simulink model "simulink_interface"  (Simulink 7.8)
settings: Solver=ode45  StartTime=0.0  StopTime=inf  RelTol=1e-3
libraries: etargetslib x7, dspnetwork x6, instrumentlib x3
settings Model: Creator=zev  LastModifiedBy=zev
settings DataIOCC: SignalLoggingSaveFormat=Dataset
settings OptimizationCC: ExpressionDepthLimit=128
settings DebuggingCC: UnderspecifiedInitializationDetection=Simplified  MergeDetectMultiDrivingBlocksExec=error  SolverPrmCheckMsg=none  FrameProcessingCompatibilityMsg=error  StateNameClashWarn=none
settings CodeAppCC: CustomSymbolStrType=$N$R$M_T
settings GRTTargetCC: TargetFunctionLibrary=NOT IN USE  CombineOutputUpdateFcns=on  CPPClassGenCompliant=on

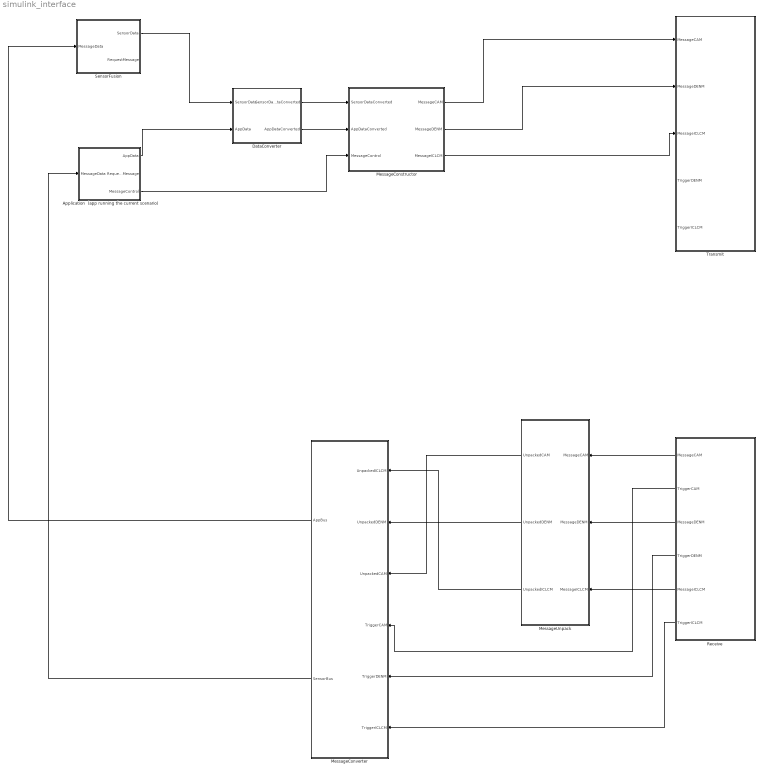
== system simulink_interface ==
  Application  (app running the current scenario) : Subsystem
  DataConverter : Subsystem
  MessageConstructor : Subsystem
  MessageConverter : Subsystem
  MessageUnpack : Subsystem
  Receive : Subsystem
  SensorFusion : Subsystem
  Transmit : Subsystem
  wires:
  Application  (app running the current scenario)/1(AppData) -> DataConverter/2(AppData)
  DataConverter/2(AppDataConverted) -> MessageConstructor/2(AppDataConverted)
  SensorFusion/1(SensorData) -> DataConverter/1(SensorData)
  DataConverter/1(SensorDataConverted) -> MessageConstructor/1(SensorDataConverted)
  MessageConstructor/1(MessageCAM) -> Transmit/1(MessageCAM)
  MessageConstructor/2(MessageDENM) -> Transmit/2(MessageDENM)
  MessageConstructor/3(MessageICLCM) -> Transmit/3(MessageICLCM)
  Application  (app running the current scenario)/3(MessageControl) -> MessageConstructor/3(MessageControl)
  Receive/1(MessageCAM) -> MessageUnpack/1(MessageCAM)
  Receive/2(TriggerCAM) -> MessageConverter/4(TriggerCAM)
  Receive/3(MessageDENM) -> MessageUnpack/2(MessageDENM)
  Receive/4(TriggerDENM) -> MessageConverter/5(TriggerDENM)
  Receive/5(MessageICLCM) -> MessageUnpack/3(MessageICLCM)
  Receive/6(TriggerICLCM) -> MessageConverter/6(TriggerICLCM)
  MessageUnpack/1(UnpackedCAM) -> MessageConverter/3(UnpackedCAM)
  MessageUnpack/2(UnpackedDENM) -> MessageConverter/2(UnpackedDENM)
  MessageConverter/1(AppBus) -> SensorFusion/1(MessageData)
  MessageConverter/2(SensorBus) -> Application  (app running the current scenario)/1(MessageData)
  MessageUnpack/3(UnpackedICLCM) -> MessageConverter/1(UnpackedICLCM)

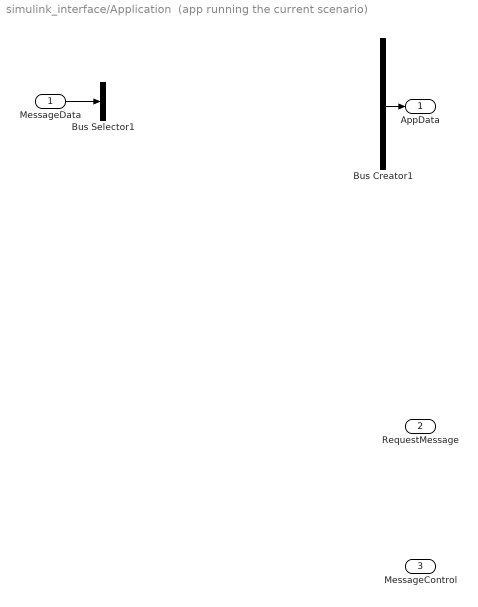
== system simulink_interface/Application  (app running the current scenario) ==
  MessageData : Inport
  Bus Creator1 : BusCreator  Inputs=26
  Bus Selector1 : BusSelector  OutputSignals=StationID,GenerationDeltaTime
  AppData : Outport
  RequestMessage : Outport  Port=2
  MessageControl : Outport  Port=3
  wires:
  MessageData/1 -> Bus Selector1/1
  Bus Creator1/1 -> AppData/1
  ? -> Bus Creator1/1  "DetectionTime"
  ? -> Bus Creator1/2  "CauseCode"
  ? -> Bus Creator1/3  "SubCauseCode"
  ? -> Bus Creator1/4  "ControllerType"
  ? -> Bus Creator1/5  "TargetLongAcc"
  ? -> Bus Creator1/6  "TimeHeadway"
  ? -> Bus Creator1/7  "CruiseSpeed"
  ? -> Bus Creator1/8  "ParticipantsReady"
  ? -> Bus Creator1/9  "StartPlatoon"
  ? -> Bus Creator1/10  "EndOfScenario"
  ? -> Bus Creator1/11  "MioId"
  ? -> Bus Creator1/12  "MioRange"
  ? -> Bus Creator1/13  "MioBearing"
  ? -> Bus Creator1/14  "MioRangeRate"
  ? -> Bus Creator1/15  "Lane"
  ? -> Bus Creator1/16  "ForwardId"
  ? -> Bus Creator1/17  "BackwardId"
  ? -> Bus Creator1/18  "MergeRequest"
  ? -> Bus Creator1/19  "SafeToMerge"
  ? -> Bus Creator1/20  "Flag"
  ? -> Bus Creator1/21  "FlagTail"
  ? -> Bus Creator1/22  "FlagHead"
  ? -> Bus Creator1/23  "PlatoonId"
  ? -> Bus Creator1/24  "DistanceTravelledCz"
  ? -> Bus Creator1/25  "Intention"
  ? -> Bus Creator1/26  "Counter"

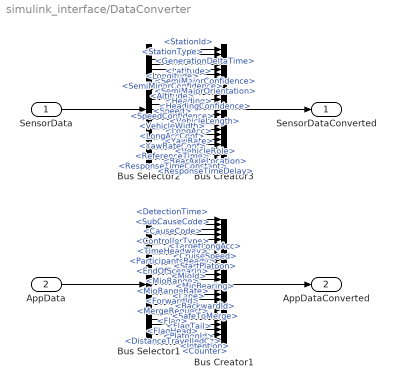
== system simulink_interface/DataConverter ==
  SensorData : Inport
  AppData : Inport  Port=2
  Bus Creator1 : BusCreator  Inputs=26
  Bus Creator3 : BusCreator  Inputs=24
  Bus Selector1 : BusSelector  OutputSignals=DetectionTime,CauseCode,SubCauseCode,ControllerType,TargetLongAcc,TimeHeadway,CruiseSpeed,ParticipantsReady,StartPlatoon,EndOfScenario,MioId,MioRange,MioBearing,MioRangeRate,Lane,ForwardId,BackwardId,MergeRequest,SafeToMerge,Flag,FlagTail,FlagHead,PlatoonId,DistanceTravelledCz,Intention,Counter
  Bus Selector2 : BusSelector  OutputSignals=StationId,GenerationDeltaTime,StationType,Latitude,Longitude,SemiMajorConfidence,SemiMinorConfidence,SemiMajorOrientation,Altitude,Heading,HeadingConfidence,Speed,SpeedConfidence,VehicleLength,VehicleWidth,LongAcc,LongAccConf,YawRate,YawRateConf,VehicleRole,ReferenceTime,RearAxleLocation,ResponseTimeConstant,ResponseTimeDelay
  SensorDataConverted : Outport
  AppDataConverted : Outport  Port=2
  wires:
  Bus Creator3/1 -> SensorDataConverted/1
  SensorData/1 -> Bus Selector2/1
  Bus Selector2/1 -> Bus Creator3/1  "<StationId>"
  Bus Selector2/2 -> Bus Creator3/2  "<GenerationDeltaTime>"
  Bus Selector2/3 -> Bus Creator3/3  "<StationType>"
  Bus Selector2/4 -> Bus Creator3/4  "<Latitude>"
  Bus Selector2/5 -> Bus Creator3/5  "<Longitude>"
  Bus Selector2/6 -> Bus Creator3/6  "<SemiMajorConfidence>"
  Bus Selector2/7 -> Bus Creator3/7  "<SemiMinorConfidence>"
  Bus Selector2/8 -> Bus Creator3/8  "<SemiMajorOrientation>"
  Bus Selector2/9 -> Bus Creator3/9  "<Altitude>"
  Bus Selector2/10 -> Bus Creator3/10  "<Heading>"
  Bus Selector2/11 -> Bus Creator3/11  "<HeadingConfidence>"
  Bus Selector2/12 -> Bus Creator3/12  "<Speed>"
  Bus Selector2/13 -> Bus Creator3/13  "<SpeedConfidence>"
  Bus Selector2/14 -> Bus Creator3/14  "<VehicleLength>"
  Bus Selector2/15 -> Bus Creator3/15  "<VehicleWidth>"
  Bus Selector2/16 -> Bus Creator3/16  "<LongAcc>"
  Bus Selector2/17 -> Bus Creator3/17  "<LongAccConf>"
  Bus Selector2/18 -> Bus Creator3/18  "<YawRate>"
  Bus Selector2/19 -> Bus Creator3/19  "<YawRateConf>"
  Bus Selector2/20 -> Bus Creator3/20  "<VehicleRole>"
  Bus Selector2/21 -> Bus Creator3/21  "<ReferenceTime>"
  Bus Selector2/22 -> Bus Creator3/22  "<RearAxleLocation>"
  Bus Selector2/23 -> Bus Creator3/23  "<ResponseTimeConstant>"
  Bus Selector2/24 -> Bus Creator3/24  "<ResponseTimeDelay>"
  Bus Creator1/1 -> AppDataConverted/1
  AppData/1 -> Bus Selector1/1
  Bus Selector1/1 -> Bus Creator1/1  "<DetectionTime>"
  Bus Selector1/2 -> Bus Creator1/2  "<CauseCode>"
  Bus Selector1/3 -> Bus Creator1/3  "<SubCauseCode>"
  Bus Selector1/4 -> Bus Creator1/4  "<ControllerType>"
  Bus Selector1/5 -> Bus Creator1/5  "<TargetLongAcc>"
  Bus Selector1/6 -> Bus Creator1/6  "<TimeHeadway>"
  Bus Selector1/7 -> Bus Creator1/7  "<CruiseSpeed>"
  Bus Selector1/8 -> Bus Creator1/8  "<ParticipantsReady>"
  Bus Selector1/9 -> Bus Creator1/9  "<StartPlatoon>"
  Bus Selector1/10 -> Bus Creator1/10  "<EndOfScenario>"
  Bus Selector1/11 -> Bus Creator1/11  "<MioId>"
  Bus Selector1/12 -> Bus Creator1/12  "<MioRange>"
  Bus Selector1/13 -> Bus Creator1/13  "<MioBearing>"
  Bus Selector1/14 -> Bus Creator1/14  "<MioRangeRate>"
  Bus Selector1/15 -> Bus Creator1/15  "<Lane>"
  Bus Selector1/16 -> Bus Creator1/16  "<ForwardId>"
  Bus Selector1/17 -> Bus Creator1/17  "<BackwardId>"
  Bus Selector1/18 -> Bus Creator1/18  "<MergeRequest>"
  Bus Selector1/19 -> Bus Creator1/19  "<SafeToMerge>"
  Bus Selector1/20 -> Bus Creator1/20  "<Flag>"
  Bus Selector1/21 -> Bus Creator1/21  "<FlagTail>"
  Bus Selector1/22 -> Bus Creator1/22  "<FlagHead>"
  Bus Selector1/23 -> Bus Creator1/23  "<PlatoonId>"
  Bus Selector1/24 -> Bus Creator1/24  "<DistanceTravelledCz>"
  Bus Selector1/25 -> Bus Creator1/25  "<Intention>"
  Bus Selector1/26 -> Bus Creator1/26  "<Counter>"

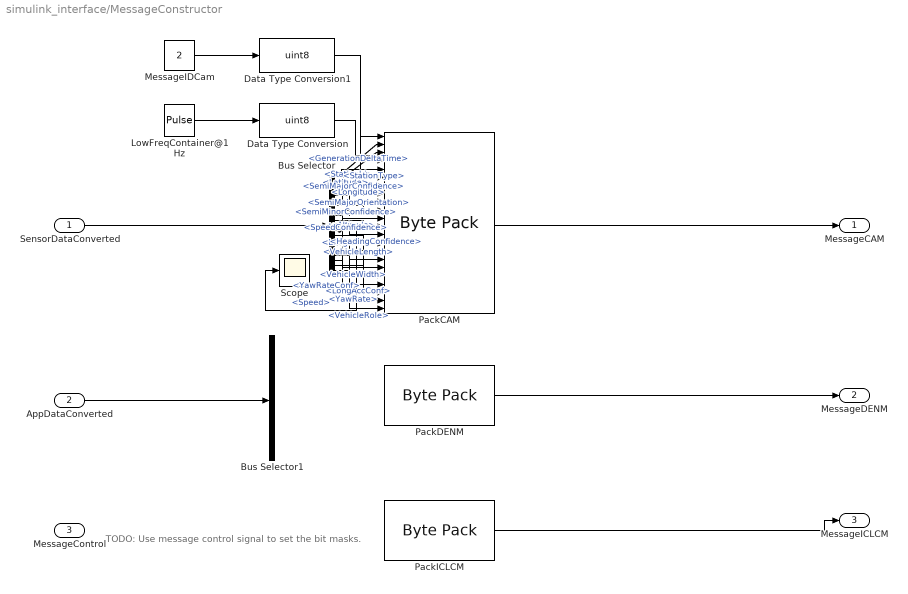
== system simulink_interface/MessageConstructor ==
  note: TODO: Use message control signal to set the bit masks.
  SensorDataConverted : Inport
  AppDataConverted : Inport  Port=2
  MessageControl : Inport  Port=3
  Bus Selector : BusSelector  OutputSignals=StationId,GenerationDeltaTime,StationType,Latitude,Longitude,SemiMajorConfidence,SemiMinorConfidence,SemiMajorOrientation,Altitude,Heading,HeadingConfidence,Speed,SpeedConfidence,VehicleLength,VehicleWidth,LongAcc,LongAccConf,YawRate,YawRateConf,VehicleRole
  Bus Selector1 : BusSelector  OutputSignals=DetectionTime,CauseCode,SubCauseCode,ControllerType,TargetLongAcc,TimeHeadway,CruiseSpeed,ParticipantsReady,StartPlatoon,EndOfScenario,MioId,MioRange,MioBearing,MioRangeRate,Lane,ForwardId,BackwardId,MergeRequest,SafeToMerge,Flag,FlagTail,FlagHead,PlatoonId,DistanceTravelledCz,Intention,Counter
  Data Type Conversion : DataTypeConversion  OutDataTypeStr=uint8
  Data Type Conversion1 : DataTypeConversion  OutDataTypeStr=uint8
  LowFreqContainer@1Hz : DiscretePulseGenerator  PulseType=Time based  Amplitude=128  Period=1  PulseWidth=0.04
  MessageIDCam : Constant  Value=2
  PackCAM : etargetslib/Byte Pack  datatypes={'uint8','int32', 'int32','uint8','int32', 'int32','int32', 'int32','int32', 'int32','int32', 'int32','int32', 'int32','int32', 'int32','int32', 'int32','int32', 'int32','int32', 'int32',}  byteAlign=1
  PackDENM : etargetslib/Byte Pack  datatypes={'int32', 'int32'}  byteAlign=1
  PackICLCM : etargetslib/Byte Pack  datatypes={'int32', 'int32'}  byteAlign=1
  Scope : Scope
      settings: SaveName=ScopeData2  DataFormat=Array
  MessageCAM : Outport
  MessageDENM : Outport  Port=2
  MessageICLCM : Outport  Port=3
  wires:
  Bus Selector/8 -> PackCAM/10  "<SemiMajorOrientation>"
  Bus Selector/4 -> PackCAM/6  "<Latitude>"
  Bus Selector/2 -> PackCAM/3  "<GenerationDeltaTime>"
  Bus Selector/9 -> PackCAM/11  "<Altitude>"
  Bus Selector/6 -> PackCAM/8  "<SemiMajorConfidence>"
  Bus Selector/7 -> PackCAM/9  "<SemiMinorConfidence>"
  Bus Selector/1 -> PackCAM/2  "<StationId>"
  PackCAM/1 -> MessageCAM/1
  Bus Selector/3 -> PackCAM/5  "<StationType>"
  Data Type Conversion/1 -> PackCAM/4
  MessageIDCam/1 -> Data Type Conversion1/1
  Bus Selector/5 -> PackCAM/7  "<Longitude>"
  Bus Selector/15 -> PackCAM/17  "<VehicleWidth>"
  Bus Selector/10 -> PackCAM/12  "<Heading>"
  Bus Selector/16 -> PackCAM/18  "<LongAcc>"
  Bus Selector/12 -> Scope/1, PackCAM/14  "<Speed>"
  Bus Selector/17 -> PackCAM/19  "<LongAccConf>"
  Bus Selector/11 -> PackCAM/13  "<HeadingConfidence>"
  Bus Selector/14 -> PackCAM/16  "<VehicleLength>"
  Bus Selector/13 -> PackCAM/15  "<SpeedConfidence>"
  SensorDataConverted/1 -> Bus Selector/1
  Data Type Conversion1/1 -> PackCAM/1
  Bus Selector/19 -> PackCAM/21  "<YawRateConf>"
  Bus Selector/20 -> PackCAM/22  "<VehicleRole>"
  LowFreqContainer@1Hz/1 -> Data Type Conversion/1
  Bus Selector/18 -> PackCAM/20  "<YawRate>"
  PackDENM/1 -> MessageDENM/1
  AppDataConverted/1 -> Bus Selector1/1
  PackICLCM/1 -> MessageICLCM/1

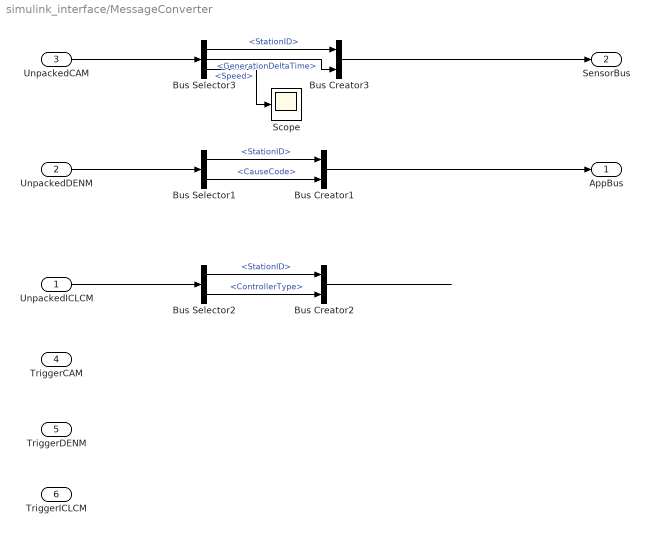
== system simulink_interface/MessageConverter ==
  UnpackedICLCM : Inport
  UnpackedDENM : Inport  Port=2
  UnpackedCAM : Inport  Port=3
  TriggerCAM : Inport  Port=4
  TriggerDENM : Inport  Port=5
  TriggerICLCM : Inport  Port=6
  Bus Creator1 : BusCreator  Inputs=2
  Bus Creator2 : BusCreator  Inputs=2
  Bus Creator3 : BusCreator  Inputs=2
  Bus Selector1 : BusSelector  OutputSignals=StationID,CauseCode
  Bus Selector2 : BusSelector  OutputSignals=StationID,ControllerType
  Bus Selector3 : BusSelector  OutputSignals=StationID,GenerationDeltaTime,Speed
  Scope : Scope
      settings: YMin=0  YMax=1.7e+07  DataFormat=Array
  AppBus : Outport
  SensorBus : Outport  Port=2
  wires:
  Bus Selector2/1 -> Bus Creator2/1  "<StationID>"
  UnpackedICLCM/1 -> Bus Selector2/1
  Bus Selector2/2 -> Bus Creator2/2  "<ControllerType>"
  Bus Creator2/1 -> ?
  Bus Selector1/1 -> Bus Creator1/1  "<StationID>"
  UnpackedDENM/1 -> Bus Selector1/1
  Bus Selector1/2 -> Bus Creator1/2  "<CauseCode>"
  Bus Creator1/1 -> AppBus/1
  Bus Selector3/1 -> Bus Creator3/1  "<StationID>"
  UnpackedCAM/1 -> Bus Selector3/1
  Bus Selector3/2 -> Bus Creator3/2  "<GenerationDeltaTime>"
  Bus Creator3/1 -> SensorBus/1
  Bus Selector3/3 -> Scope/1  "<Speed>"

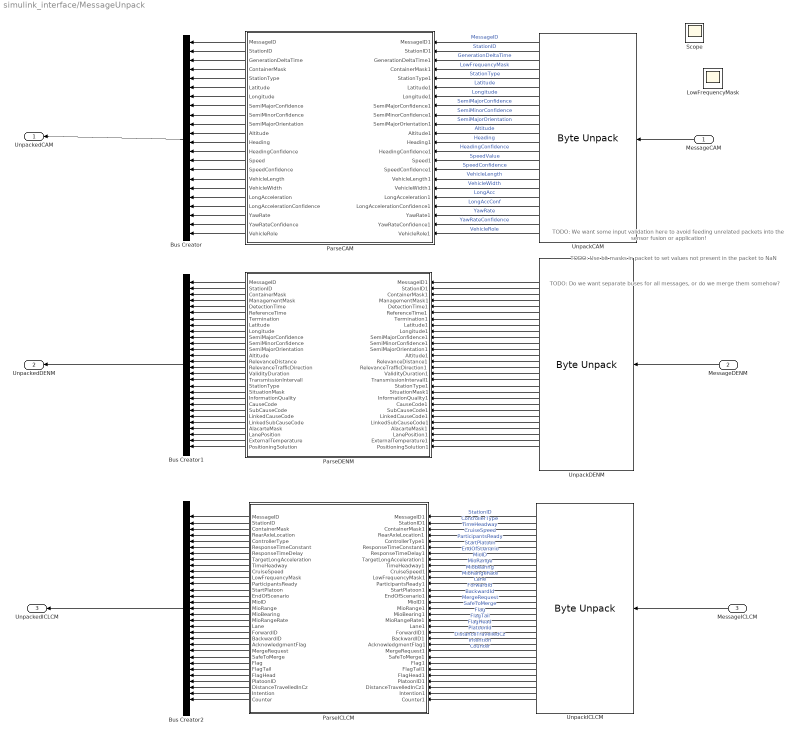
== system simulink_interface/MessageUnpack ==
  note: TODO: Do we want separate buses for all messages, or do we merge them somehow?
  note: TODO: Use bit masks in packet to set values not present in the packet to NaN
  note: TODO: We want some input validation here to avoid feeding unrelated packets
      | into the sensor fusion or application!
  MessageCAM : Inport
  MessageDENM : Inport  Port=2
  MessageICLCM : Inport  Port=3
  Bus Creator : BusCreator  Inputs=22
  Bus Creator1 : BusCreator  Inputs=28
  Bus Creator2 : BusCreator  Inputs=31
  LowFrequencyMask : Scope
      settings: DataFormat=Array
  ParseCAM : MATLAB Function  TreatAsAtomicUnit=on
  ParseDENM : MATLAB Function  TreatAsAtomicUnit=on
  ParseICLCM : MATLAB Function  TreatAsAtomicUnit=on
  Scope : Scope
      settings: SaveName=ScopeData3  DataFormat=Array
  UnpackCAM : etargetslib/Byte Unpack  dimensions={[1],[1],[1],[1],[1],[1],[1],[1],[1],[1],[1],[1],[1],[1],[1],[1],[1],[1],[1],[1],[1],[1],}  datatypes={'uint8','int32', 'int32','uint8','int32', 'int32','int32', 'int32','int32', 'int32','int32', 'int32','int32', 'int32','int32', 'int32','int32', 'int32','int32', 'int32','int32', 'int32',}  byteAlign=1
  UnpackDENM : etargetslib/Byte Unpack  dimensions={[1], [1], [1], [1], [1], [1], [1], [1], [1], [1], [1], [1], [1], [1], [1], [1], [1], [1], [1], [1], [1], [1], [1], [1], [1], [1], [1], [1]}  datatypes="{'uint8', 'int32', 'uint8',  'uint8', 'int32', 'int32', 'int32', 'int32', 'int32',  'int32', 'int32', 'int32', 'int32', 'int32', 'int32', 'int32', 'int32', 'int32', 'uint8',  'int32', 'int32', 'int32', 'int32', 'int32', 'uint8',  'int32', 'int32', 'int32'}"  byteAlign=1
  UnpackICLCM : etargetslib/Byte Unpack  dimensions={[1],[1], [1],[1], [1],[1], [1],[1], [1],[1], [1],[1], [1],[1], [1],[1], [1],[1],[1],[1], [1],[1], [1],[1],[1],[1],[1],[1], [1],[1], [1]}  datatypes={'uint8', 'int32', 'uint8', 'int32', 'int32','int32', 'int32','int32', 'int32','int32', 'uint8', 'int32','int32', 'int32','int32', 'int32','int32', 'int32','int32', 'int32','int32', 'int32','int32', 'int32','int32', 'int32', 'uint32', 'int32','int32', 'int32', 'uint32'}  byteAlign=1
  UnpackedCAM : Outport
  UnpackedDENM : Outport  Port=2
  UnpackedICLCM : Outport  Port=3
  wires:
  UnpackCAM/4 -> ParseCAM/4(ContainerMask1)  "LowFrequencyMask"
  UnpackCAM/10 -> ParseCAM/10(SemiMajorOrientation1)  "SemiMajorOrientation"
  UnpackCAM/11 -> ParseCAM/11(Altitude1)  "Altitude"
  UnpackCAM/9 -> ParseCAM/9(SemiMinorConfidence1)  "SemiMinorConfidence"
  UnpackCAM/7 -> ParseCAM/7(Longitude1)  "Longitude"
  UnpackCAM/8 -> ParseCAM/8(SemiMajorConfidence1)  "SemiMajorConfidence"
  UnpackCAM/6 -> ParseCAM/6(Latitude1)  "Latitude"
  UnpackCAM/5 -> ParseCAM/5(StationType1)  "StationType"
  UnpackCAM/3 -> ParseCAM/3(GenerationDeltaTime1)  "GenerationDeltaTime"
  MessageCAM/1 -> UnpackCAM/1
  MessageDENM/1 -> UnpackDENM/1
  MessageICLCM/1 -> UnpackICLCM/1
  Bus Creator1/1 -> UnpackedDENM/1
  Bus Creator2/1 -> UnpackedICLCM/1
  Bus Creator/1 -> UnpackedCAM/1
  UnpackCAM/2 -> ParseCAM/2(StationID1)  "StationID"
  UnpackCAM/1 -> ParseCAM/1(MessageID1)  "MessageID"
  UnpackCAM/21 -> ParseCAM/21(YawRateConfidence1)  "YawRateConfidence"
  UnpackCAM/22 -> ParseCAM/22(VehicleRole1)  "VehicleRole"
  UnpackCAM/12 -> ParseCAM/12(Heading1)  "Heading"
  UnpackCAM/13 -> ParseCAM/13(HeadingConfidence1)  "HeadingConfidence"
  UnpackCAM/14 -> ParseCAM/14(Speed1)  "SpeedValue"
  UnpackCAM/15 -> ParseCAM/15(SpeedConfidence1)  "SpeedConfidence"
  UnpackCAM/16 -> ParseCAM/16(VehicleLength1)  "VehicleLength"
  UnpackCAM/17 -> ParseCAM/17(VehicleWidth1)  "VehicleWidth"
  UnpackCAM/18 -> ParseCAM/18(LongAcceleration1)  "LongAcc"
  UnpackCAM/19 -> ParseCAM/19(LongAccelerationConfidence1)  "LongAccConf"
  UnpackCAM/20 -> ParseCAM/20(YawRate1)  "YawRate"
  ParseCAM/1(MessageID) -> Bus Creator/1
  ParseCAM/22(VehicleRole) -> Bus Creator/22
  ParseCAM/2(StationID) -> Bus Creator/2
  ParseCAM/3(GenerationDeltaTime) -> Bus Creator/3
  ParseCAM/4(ContainerMask) -> Bus Creator/4
  ParseCAM/5(StationType) -> Bus Creator/5
  ParseCAM/6(Latitude) -> Bus Creator/6
  ParseCAM/7(Longitude) -> Bus Creator/7
  ParseCAM/8(SemiMajorConfidence) -> Bus Creator/8
  ParseCAM/9(SemiMinorConfidence) -> Bus Creator/9
  ParseCAM/10(SemiMajorOrientation) -> Bus Creator/10
  ParseCAM/11(Altitude) -> Bus Creator/11
  ParseCAM/12(Heading) -> Bus Creator/12
  ParseCAM/13(HeadingConfidence) -> Bus Creator/13
  ParseCAM/14(Speed) -> Bus Creator/14
  ParseCAM/15(SpeedConfidence) -> Bus Creator/15
  ParseCAM/16(VehicleLength) -> Bus Creator/16
  ParseCAM/17(VehicleWidth) -> Bus Creator/17
  ParseCAM/18(LongAcceleration) -> Bus Creator/18
  ParseCAM/19(LongAccelerationConfidence) -> Bus Creator/19
  ParseCAM/20(YawRate) -> Bus Creator/20
  ParseCAM/21(YawRateConfidence) -> Bus Creator/21
  UnpackDENM/1 -> ParseDENM/1(MessageID1)
  UnpackDENM/2 -> ParseDENM/2(StationID1)
  UnpackDENM/3 -> ParseDENM/3(ContainerMask1)
  UnpackDENM/4 -> ParseDENM/4(ManagementMask1)
  UnpackDENM/5 -> ParseDENM/5(DetectionTime1)
  UnpackDENM/6 -> ParseDENM/6(ReferenceTime1)
  UnpackDENM/7 -> ParseDENM/7(Termination1)
  UnpackDENM/8 -> ParseDENM/8(Latitude1)
  UnpackDENM/9 -> ParseDENM/9(Longitude1)
  UnpackDENM/10 -> ParseDENM/10(SemiMajorConfidence1)
  UnpackDENM/11 -> ParseDENM/11(SemiMinorConfidence1)
  UnpackDENM/12 -> ParseDENM/12(SemiMajorOrientation1)
  UnpackDENM/13 -> ParseDENM/13(Altitude1)
  UnpackDENM/14 -> ParseDENM/14(RelevanceDistance1)
  UnpackDENM/15 -> ParseDENM/15(RelevanceTrafficDirection1)
  UnpackDENM/16 -> ParseDENM/16(ValidityDuration1)
  UnpackDENM/17 -> ParseDENM/17(TransmissionIntervall1)
  UnpackDENM/18 -> ParseDENM/18(StationType1)
  UnpackDENM/19 -> ParseDENM/19(SituationMask1)
  UnpackDENM/20 -> ParseDENM/20(InformationQuality1)
  UnpackDENM/21 -> ParseDENM/21(CauseCode1)
  UnpackDENM/22 -> ParseDENM/22(SubCauseCode1)
  UnpackDENM/23 -> ParseDENM/23(LinkedCauseCode1)
  UnpackDENM/24 -> ParseDENM/24(LinkedSubCauseCode1)
  UnpackDENM/25 -> ParseDENM/25(AlacarteMask1)
  UnpackDENM/26 -> ParseDENM/26(LanePosition1)
  UnpackDENM/27 -> ParseDENM/27(ExternalTemperature1)
  UnpackDENM/28 -> ParseDENM/28(PositioningSolution1)
  ParseDENM/1(MessageID) -> Bus Creator1/1
  ParseDENM/2(StationID) -> Bus Creator1/2
  ParseDENM/3(ContainerMask) -> Bus Creator1/3
  ParseDENM/4(ManagementMask) -> Bus Creator1/4
  ParseDENM/5(DetectionTime) -> Bus Creator1/5
  ParseDENM/6(ReferenceTime) -> Bus Creator1/6
  ParseDENM/7(Termination) -> Bus Creator1/7
  ParseDENM/8(Latitude) -> Bus Creator1/8
  ParseDENM/9(Longitude) -> Bus Creator1/9
  ParseDENM/10(SemiMajorConfidence) -> Bus Creator1/10
  ParseDENM/11(SemiMinorConfidence) -> Bus Creator1/11
  ParseDENM/12(SemiMajorOrientation) -> Bus Creator1/12
  ParseDENM/13(Altitude) -> Bus Creator1/13
  ParseDENM/14(RelevanceDistance) -> Bus Creator1/14
  ParseDENM/15(RelevanceTrafficDirection) -> Bus Creator1/15
  ParseDENM/16(ValidityDuration) -> Bus Creator1/16
  ParseDENM/17(TransmissionIntervall) -> Bus Creator1/17
  ParseDENM/18(StationType) -> Bus Creator1/18
  ParseDENM/19(SituationMask) -> Bus Creator1/19
  ParseDENM/20(InformationQuality) -> Bus Creator1/20
  ParseDENM/21(CauseCode) -> Bus Creator1/21
  ParseDENM/22(SubCauseCode) -> Bus Creator1/22
  ParseDENM/23(LinkedCauseCode) -> Bus Creator1/23
  ParseDENM/24(LinkedSubCauseCode) -> Bus Creator1/24
  ParseDENM/25(AlacarteMask) -> Bus Creator1/25
  ParseDENM/26(LanePosition) -> Bus Creator1/26
  ParseDENM/27(ExternalTemperature) -> Bus Creator1/27
  ParseDENM/28(PositioningSolution) -> Bus Creator1/28
  UnpackICLCM/1 -> ParseICLCM/1(MessageID1)  "StationID"
  UnpackICLCM/2 -> ParseICLCM/2(StationID1)  "ControllerType"
  UnpackICLCM/3 -> ParseICLCM/3(ContainerMask1)  "TimeHeadway"
  UnpackICLCM/4 -> ParseICLCM/4(RearAxleLocation1)  "CruiseSpeed"
  UnpackICLCM/5 -> ParseICLCM/5(ControllerType1)  "ParticipantsReady"
  UnpackICLCM/6 -> ParseICLCM/6(ResponseTimeConstant1)  "StartPlatoon"
  UnpackICLCM/7 -> ParseICLCM/7(ResponseTimeDelay1)  "EndOfScenario"
  UnpackICLCM/8 -> ParseICLCM/8(TargetLongAcceleration1)  "MioID"
  UnpackICLCM/9 -> ParseICLCM/9(TimeHeadway1)  "MioRange"
  UnpackICLCM/10 -> ParseICLCM/10(CruiseSpeed1)  "MioBearing"
  UnpackICLCM/11 -> ParseICLCM/11(LowFrequencyMask1)  "MioRangeRate"
  UnpackICLCM/12 -> ParseICLCM/12(ParticipantsReady1)  "Lane"
  UnpackICLCM/13 -> ParseICLCM/13(StartPlatoon1)  "ForwardId"
  UnpackICLCM/14 -> ParseICLCM/14(EndOfScenario1)  "BackwardId"
  UnpackICLCM/15 -> ParseICLCM/15(MioID1)  "MergeRequest"
  UnpackICLCM/16 -> ParseICLCM/16(MioRange1)  "SafeToMerge"
  UnpackICLCM/17 -> ParseICLCM/17(MioBearing1)  "Flag"
  UnpackICLCM/18 -> ParseICLCM/18(MioRangeRate1)  "FlagTail"
  UnpackICLCM/19 -> ParseICLCM/19(Lane1)  "FlagHead"
  UnpackICLCM/20 -> ParseICLCM/20(ForwardID1)  "PlatoonId"
  UnpackICLCM/21 -> ParseICLCM/21(BackwardID1)  "DistanceTravelledCz"
  UnpackICLCM/22 -> ParseICLCM/22(AcknowledgmentFlag1)  "Intention"
  UnpackICLCM/23 -> ParseICLCM/23(MergeRequest1)  "Counter"
  UnpackICLCM/24 -> ParseICLCM/24(SafeToMerge1)
  UnpackICLCM/25 -> ParseICLCM/25(Flag1)
  UnpackICLCM/26 -> ParseICLCM/26(FlagTail1)
  UnpackICLCM/27 -> ParseICLCM/27(FlagHead1)
  UnpackICLCM/28 -> ParseICLCM/28(PlatoonID1)
  UnpackICLCM/29 -> ParseICLCM/29(DistanceTravelledInCz1)
  UnpackICLCM/30 -> ParseICLCM/30(Intention1)
  UnpackICLCM/31 -> ParseICLCM/31(Counter1)
  ParseICLCM/1(MessageID) -> Bus Creator2/1
  ParseICLCM/2(StationID) -> Bus Creator2/2
  ParseICLCM/3(ContainerMask) -> Bus Creator2/3
  ParseICLCM/4(RearAxleLocation) -> Bus Creator2/4
  ParseICLCM/5(ControllerType) -> Bus Creator2/5
  ParseICLCM/6(ResponseTimeConstant) -> Bus Creator2/6
  ParseICLCM/7(ResponseTimeDelay) -> Bus Creator2/7
  ParseICLCM/8(TargetLongAcceleration) -> Bus Creator2/8
  ParseICLCM/9(TimeHeadway) -> Bus Creator2/9
  ParseICLCM/10(CruiseSpeed) -> Bus Creator2/10
  ParseICLCM/11(LowFrequencyMask) -> Bus Creator2/11
  ParseICLCM/12(ParticipantsReady) -> Bus Creator2/12
  ParseICLCM/13(StartPlatoon) -> Bus Creator2/13
  ParseICLCM/14(EndOfScenario) -> Bus Creator2/14
  ParseICLCM/15(MioID) -> Bus Creator2/15
  ParseICLCM/16(MioRange) -> Bus Creator2/16
  ParseICLCM/17(MioBearing) -> Bus Creator2/17
  ParseICLCM/18(MioRangeRate) -> Bus Creator2/18
  ParseICLCM/19(Lane) -> Bus Creator2/19
  ParseICLCM/20(ForwardID) -> Bus Creator2/20
  ParseICLCM/21(BackwardID) -> Bus Creator2/21
  ParseICLCM/22(AcknowledgmentFlag) -> Bus Creator2/22
  ParseICLCM/23(MergeRequest) -> Bus Creator2/23
  ParseICLCM/24(SafeToMerge) -> Bus Creator2/24
  ParseICLCM/25(Flag) -> Bus Creator2/25
  ParseICLCM/26(FlagTail) -> Bus Creator2/26
  ParseICLCM/27(FlagHead) -> Bus Creator2/27
  ParseICLCM/28(PlatoonID) -> Bus Creator2/28
  ParseICLCM/29(DistanceTravelledInCz) -> Bus Creator2/29
  ParseICLCM/30(Intention) -> Bus Creator2/30
  ParseICLCM/31(Counter) -> Bus Creator2/31

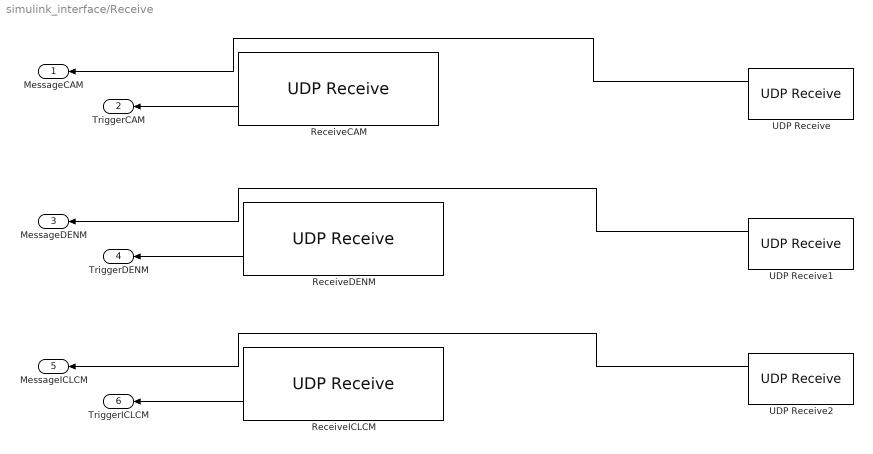
== system simulink_interface/Receive ==
  ReceiveCAM : instrumentlib/UDP Receive  Host=127.0.0.1  Port=4000  LocalPort=-1  DataSize="[1  82]"  EnableBlockingMode=off  Timeout=10  SampleTime=0.01  DataType=uint8  ByteOrder=BigEndian
  ReceiveDENM : instrumentlib/UDP Receive  Host=0.0.0.0  Port=4001  LocalPort=-1  DataSize="[1  12]"  EnableBlockingMode=off  Timeout=10  SampleTime=0.01  DataType=uint8  ByteOrder=BigEndian
  ReceiveICLCM : instrumentlib/UDP Receive  Host=0.0.0.0  Port=4002  LocalPort=-1  DataSize="[1  92]"  EnableBlockingMode=off  Timeout=10  SampleTime=0.01  DataType=uint8  ByteOrder=BigEndian
  UDP Receive : dspnetwork/UDP Receive  localURL='0.0.0.0'  localPort=5000  remoteURL='0.0.0.0'  remotePort=-1  recvBufferSize=8192  dims=82  signalDatatype=uint8  isVarSize=off  showBlockingTime=off  blockingTime=0  sampletime=0.04
  UDP Receive1 : dspnetwork/UDP Receive  localURL='0.0.0.0'  localPort=5001  remoteURL='0.0.0.0'  remotePort=-1  recvBufferSize=8192  dims=97  signalDatatype=uint8  isVarSize=off  showBlockingTime=off  blockingTime=0  sampletime=0.04
  UDP Receive2 : dspnetwork/UDP Receive  localURL='0.0.0.0'  localPort=5002  remoteURL='0.0.0.0'  remotePort=-1  recvBufferSize=8192  dims=115  signalDatatype=uint8  isVarSize=off  showBlockingTime=off  blockingTime=0  sampletime=0.04
  MessageCAM : Outport
  TriggerCAM : Outport  Port=2
  MessageDENM : Outport  Port=3
  TriggerDENM : Outport  Port=4
  MessageICLCM : Outport  Port=5
  TriggerICLCM : Outport  Port=6
  wires:
  UDP Receive/1 -> MessageCAM/1
  ReceiveICLCM/2 -> TriggerICLCM/1
  UDP Receive2/1 -> MessageICLCM/1
  ReceiveDENM/2 -> TriggerDENM/1
  UDP Receive1/1 -> MessageDENM/1
  ReceiveCAM/2 -> TriggerCAM/1

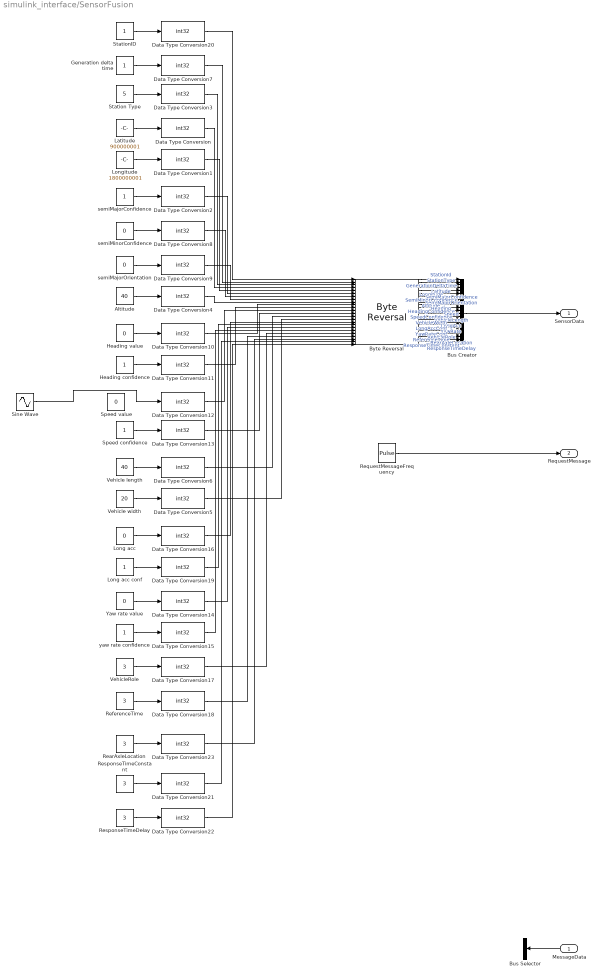
== system simulink_interface/SensorFusion ==
  MessageData : Inport
  Altitude : Constant  Value=40
  Bus Creator : BusCreator  Inputs=24
  Bus Selector : BusSelector  OutputSignals=StationID
  Byte Reversal : etargetslib/Byte Reversal  numInp=24
  Data Type Conversion{,1..23} (24 alike) : DataTypeConversion  OutDataTypeStr=int32
  Generation delta time : Constant
  Heading confidence : Constant
  Heading value : Constant  Value=0
  Latitude : Constant  Value=900000001
  Long acc : Constant  Value=0
  Long acc conf : Constant
  Longitude : Constant  Value=1800000001
  RearAxleLocation : Constant  Value=3
  ReferenceTime : Constant  Value=3
  RequestMessageFrequency : DiscretePulseGenerator  PulseType=Time based  Period=0.01  PulseWidth=5
  ResponseTimeConstant : Constant  Value=3
  ResponseTimeDelay : Constant  Value=3
  Sine Wave : Sin  Bias=1  Frequency=100  SampleTime=0
  Speed confidence : Constant
  Speed value : Constant  Value=0
  Station Type : Constant  Value=5
  StationID : Constant
  Vehicle length : Constant  Value=40
  Vehicle width : Constant  Value=20
  VehicleRole : Constant  Value=3
  Yaw rate value : Constant  Value=0
  "semiMajorConfidence " : Constant
  "semiMajorOrientation " : Constant  Value=0
  "semiMinorConfidence " : Constant  Value=0
  yaw rate confidence : Constant
  SensorData : Outport
  RequestMessage : Outport  Port=2
  wires:
  Bus Creator/1 -> SensorData/1
  Station Type/1 -> Data Type Conversion3/1
  Generation delta time/1 -> Data Type Conversion7/1
  yaw rate confidence/1 -> Data Type Conversion15/1
  Long acc/1 -> Data Type Conversion16/1
  VehicleRole/1 -> Data Type Conversion17/1
  Long acc conf/1 -> Data Type Conversion19/1
  ReferenceTime/1 -> Data Type Conversion18/1
  Vehicle length/1 -> Data Type Conversion6/1
  Vehicle width/1 -> Data Type Conversion5/1
  Latitude/1 -> Data Type Conversion/1
  Longitude/1 -> Data Type Conversion1/1
  "semiMajorConfidence "/1 -> Data Type Conversion2/1
  "semiMinorConfidence "/1 -> Data Type Conversion8/1
  "semiMajorOrientation "/1 -> Data Type Conversion9/1
  Heading confidence/1 -> Data Type Conversion11/1
  Heading value/1 -> Data Type Conversion10/1
  Sine Wave/1 -> Data Type Conversion12/1
  Speed confidence/1 -> Data Type Conversion13/1
  Yaw rate value/1 -> Data Type Conversion14/1
  StationID/1 -> Data Type Conversion20/1
  Altitude/1 -> Data Type Conversion4/1
  ResponseTimeConstant/1 -> Data Type Conversion21/1
  ResponseTimeDelay/1 -> Data Type Conversion22/1
  RearAxleLocation/1 -> Data Type Conversion23/1
  Data Type Conversion20/1 -> Byte Reversal/1
  Data Type Conversion7/1 -> Byte Reversal/2
  Data Type Conversion3/1 -> Byte Reversal/3
  Data Type Conversion/1 -> Byte Reversal/4
  Data Type Conversion1/1 -> Byte Reversal/5
  Data Type Conversion2/1 -> Byte Reversal/6
  Data Type Conversion8/1 -> Byte Reversal/7
  Data Type Conversion9/1 -> Byte Reversal/8
  Data Type Conversion4/1 -> Byte Reversal/9
  Data Type Conversion10/1 -> Byte Reversal/10
  Data Type Conversion11/1 -> Byte Reversal/11
  Data Type Conversion12/1 -> Byte Reversal/12
  Data Type Conversion13/1 -> Byte Reversal/13
  Data Type Conversion6/1 -> Byte Reversal/14
  Data Type Conversion5/1 -> Byte Reversal/15
  Data Type Conversion16/1 -> Byte Reversal/16
  Data Type Conversion19/1 -> Byte Reversal/17
  Data Type Conversion14/1 -> Byte Reversal/18
  Data Type Conversion15/1 -> Byte Reversal/19
  Data Type Conversion17/1 -> Byte Reversal/20
  Data Type Conversion18/1 -> Byte Reversal/21
  Data Type Conversion23/1 -> Byte Reversal/22
  Data Type Conversion21/1 -> Byte Reversal/23
  Data Type Conversion22/1 -> Byte Reversal/24
  Byte Reversal/1 -> Bus Creator/1  "StationId"
  Byte Reversal/2 -> Bus Creator/2  "GenerationDeltaTime"
  Byte Reversal/3 -> Bus Creator/3  "StationType"
  Byte Reversal/4 -> Bus Creator/4  "Latitude"
  Byte Reversal/5 -> Bus Creator/5  "Longitude"
  Byte Reversal/6 -> Bus Creator/6  "SemiMajorConfidence"
  Byte Reversal/7 -> Bus Creator/7  "SemiMinorConfidence"
  Byte Reversal/8 -> Bus Creator/8  "SemiMajorOrientation"
  Byte Reversal/9 -> Bus Creator/9  "Altitude"
  Byte Reversal/10 -> Bus Creator/10  "Heading"
  Byte Reversal/11 -> Bus Creator/11  "HeadingConfidence"
  Byte Reversal/12 -> Bus Creator/12  "Speed"
  Byte Reversal/13 -> Bus Creator/13  "SpeedConfidence"
  Byte Reversal/14 -> Bus Creator/14  "VehicleLength"
  Byte Reversal/15 -> Bus Creator/15  "VehicleWidth"
  Byte Reversal/16 -> Bus Creator/16  "LongAcc"
  Byte Reversal/17 -> Bus Creator/17  "LongAccConf"
  Byte Reversal/18 -> Bus Creator/18  "YawRate"
  Byte Reversal/19 -> Bus Creator/19  "YawRateConf"
  Byte Reversal/20 -> Bus Creator/20  "VehicleRole"
  Byte Reversal/21 -> Bus Creator/21  "ReferenceTime"
  Byte Reversal/22 -> Bus Creator/22  "RearAxleLocation"
  Byte Reversal/23 -> Bus Creator/23  "ResponseTimeConstant"
  Byte Reversal/24 -> Bus Creator/24  "ResponseTimeDelay"
  RequestMessageFrequency/1 -> RequestMessage/1
  MessageData/1 -> Bus Selector/1

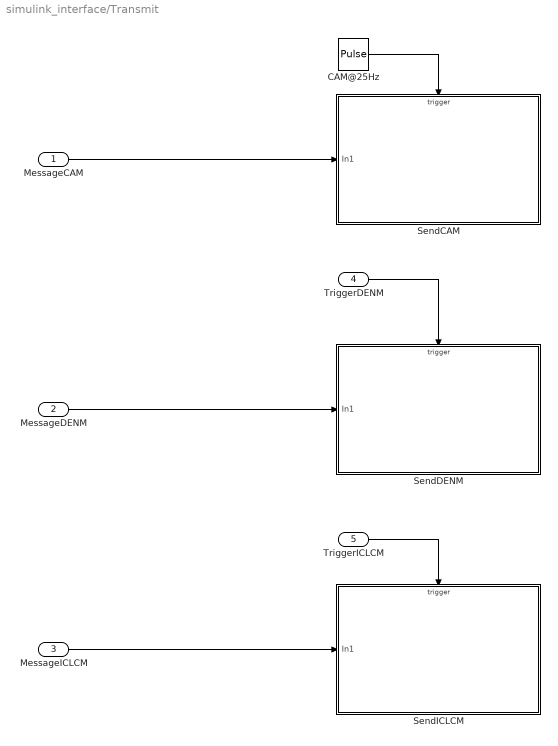
== system simulink_interface/Transmit ==
  MessageCAM : Inport
  MessageDENM : Inport  Port=2
  MessageICLCM : Inport  Port=3
  TriggerDENM : Inport  Port=4
  TriggerICLCM : Inport  Port=5
  CAM@25Hz : DiscretePulseGenerator  PulseType=Time based  Period=0.04  PulseWidth=5
  SendCAM : Subsystem
  SendDENM : Subsystem
  SendICLCM : Subsystem
  wires:
  MessageDENM/1 -> SendDENM/1(In1)
  MessageICLCM/1 -> SendICLCM/1(In1)
  TriggerDENM/1 -> SendDENM/Trigger
  TriggerICLCM/1 -> SendICLCM/Trigger
  CAM@25Hz/1 -> SendCAM/Trigger
  MessageCAM/1 -> SendCAM/1(In1)

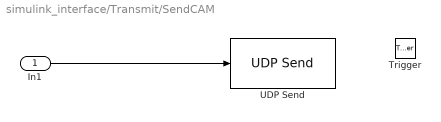
== system simulink_interface/Transmit/SendCAM ==
  In1 : Inport
  Trigger : TriggerPort  PortDimensions=1
  UDP Send : dspnetwork/UDP Send  remoteURL='127.0.0.1'  remotePort=5000  localURL='0.0.0.0'  localPortSource=Automatically determine  localPort=-1  sampletime=-1  separateLengthPort=0
  wires:
  In1/1 -> UDP Send/1

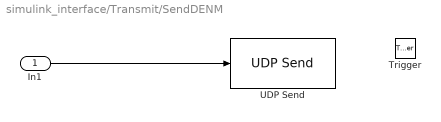
== system simulink_interface/Transmit/SendDENM ==
  In1 : Inport
  Trigger : TriggerPort  PortDimensions=1
  UDP Send : dspnetwork/UDP Send  remoteURL='127.0.0.1'  remotePort=5001  localURL='0.0.0.0'  localPortSource=Automatically determine  localPort=-1  sampletime=-1  separateLengthPort=0
  wires:
  In1/1 -> UDP Send/1

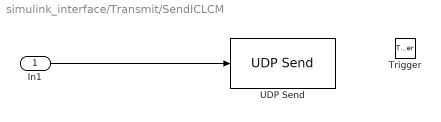
== system simulink_interface/Transmit/SendICLCM ==
  In1 : Inport
  Trigger : TriggerPort  PortDimensions=1
  UDP Send : dspnetwork/UDP Send  remoteURL='127.0.0.1'  remotePort=5001  localURL='0.0.0.0'  localPortSource=Automatically determine  localPort=-1  sampletime=-1  separateLengthPort=0
  wires:
  In1/1 -> UDP Send/1

== matlab function MessageUnpack/ParseDENM ==
  data: MessageID1 input double; MessageID output double; StationID1 input double; ContainerMask1 input double; ManagementMask1 input double; DetectionTime1 input double; ReferenceTime1 input double; Termination1 input double; Latitude1 input double; Longitude1 input double; SemiMajorConfidence1 input double; SemiMinorConfidence1 input double; SemiMajorOrientation1 input double; Altitude1 input double; RelevanceDistance1 input double; RelevanceTrafficDirection1 input double; ValidityDuration1 input double; TransmissionIntervall1 input double; StationType1 input double; SituationMask1 input double; InformationQuality1 input double; CauseCode1 input double; SubCauseCode1 input double; LinkedCauseCode1 input double; LinkedSubCauseCode1 input double; AlacarteMask1 input double; LanePosition1 input double; ExternalTemperature1 input double; PositioningSolution1 input double; StationID output double; ContainerMask output double; ManagementMask output double; DetectionTime output double; ReferenceTime output double; Termination output double; Latitude output double; Longitude output double; SemiMajorConfidence output double; SemiMinorConfidence output double; SemiMajorOrientation output double; Altitude output double; RelevanceDistance output double; RelevanceTrafficDirection output double; ValidityDuration output double; TransmissionIntervall output double; StationType output double; SituationMask output double; InformationQuality output double; CauseCode output double; SubCauseCode output double; LinkedCauseCode output double; LinkedSubCauseCode output double; AlacarteMask output double; LanePosition output double; ExternalTemperature output double; PositioningSolution output double
function [MessageID, StationID, ContainerMask, ManagementMask, DetectionTime, ReferenceTime, Termination, Latitude, Longitude, SemiMajorConfidence, SemiMinorConfidence, SemiMajorOrientation, Altitude, RelevanceDistance, RelevanceTrafficDirection, ValidityDuration, TransmissionIntervall, StationType, SituationMask, InformationQuality, CauseCode, SubCauseCode, LinkedCauseCode, LinkedSubCauseCode, AlacarteMask, LanePosition, ExternalTemperature, PositioningSolution] = parseDENM(MessageID1, StationID1, ContainerMask1, ManagementMask1, DetectionTime1, ReferenceTime1, Termination1, Latitude1, Longitude1, SemiMajorConfidence1, SemiMinorConfidence1, SemiMajorOrientation1, Altitude1, RelevanceDistance1, RelevanceTrafficDirection1, ValidityDuration1, TransmissionIntervall1, StationType1, SituationMask1, InformationQuality1, CauseCode1, SubCauseCode1, LinkedCauseCode1, LinkedSubCauseCode1, AlacarteMask1, LanePosition1, ExternalTemperature1, PositioningSolution1)
%parseDENM - Parses a local DENM message.



MessageID = MessageID1;
StationID = StationID1;
ContainerMask = ContainerMask1;
ManagementMask = ManagementMask1;
DetectionTime = DetectionTime1;
ReferenceTime = ReferenceTime1;
Termination = Termination1;
Latitude = Latitude1;
Longitude = Longitude1; 
SemiMajorConfidence = SemiMajorConfidence1;
SemiMinorConfidence = SemiMinorConfidence1; 
SemiMajorOrientation = SemiMajorOrientation1;
Altitude = Altitude1; 
RelevanceDistance = RelevanceDistance1;
RelevanceTrafficDirection = RelevanceTrafficDirection1; 
ValidityDuration = ValidityDuration1; 
TransmissionIntervall = TransmissionIntervall1; 
StationType = StationType1; 
SituationMask = SituationMask1; 
InformationQuality = InformationQuality1; 
CauseCode = CauseCode1; 
SubCauseCode = SubCauseCode1; 
LinkedCauseCode = LinkedCauseCode1; 
LinkedSubCauseCode = LinkedSubCauseCode1; 
AlacarteMask = AlacarteMask1;
LanePosition = LanePosition1;
ExternalTemperature = ExternalTemperature1; 
PositioningSolution = PositioningSolution1;

== matlab function MessageUnpack/ParseCAM ==
  data: MessageID output double; MessageID1 input double; StationID output double; GenerationDeltaTime output double; ContainerMask output double; StationType output double; Latitude output double; Longitude output double; SemiMajorConfidence output double; SemiMinorConfidence output double; SemiMajorOrientation output double; Altitude output double; Heading output double; HeadingConfidence output double; Speed output double; SpeedConfidence output double; VehicleLength output double; VehicleWidth output double; LongAcceleration output double; LongAccelerationConfidence output double; YawRate output double; YawRateConfidence output double; VehicleRole output double; StationID1 input double; GenerationDeltaTime1 input double; ContainerMask1 input double; StationType1 input double; Latitude1 input double; Longitude1 input double; SemiMajorConfidence1 input double; SemiMinorConfidence1 input double; SemiMajorOrientation1 input double; Altitude1 input double; Heading1 input double; HeadingConfidence1 input double; Speed1 input double; SpeedConfidence1 input double; VehicleLength1 input double; VehicleWidth1 input double; LongAcceleration1 input double; LongAccelerationConfidence1 input double; YawRate1 input double; YawRateConfidence1 input double; VehicleRole1 input double
function [MessageID, StationID, GenerationDeltaTime, ContainerMask, StationType, Latitude, Longitude, SemiMajorConfidence, SemiMinorConfidence, SemiMajorOrientation, Altitude, Heading, HeadingConfidence, Speed, SpeedConfidence, VehicleLength, VehicleWidth, LongAcceleration, LongAccelerationConfidence, YawRate, YawRateConfidence, VehicleRole] = parseCAM(MessageID1, StationID1, GenerationDeltaTime1, ContainerMask1, StationType1, Latitude1, Longitude1, SemiMajorConfidence1, SemiMinorConfidence1, SemiMajorOrientation1, Altitude1, Heading1, HeadingConfidence1, Speed1, SpeedConfidence1, VehicleLength1, VehicleWidth1, LongAcceleration1, LongAccelerationConfidence1, YawRate1, YawRateConfidence1, VehicleRole1)
%parseCAM - Parses a local CAM message. Used to do some conversion in order
%to make the values compatible with the Simulink model.

MessageID = MessageID1;
StationID = StationID1;
GenerationDeltaTime = GenerationDeltaTime1;
ContainerMask = ContainerMask1;
StationType = StationType1;
Latitude = Latitude1;
Longitude = Longitude1;
SemiMajorConfidence = SemiMajorConfidence1;
SemiMinorConfidence = SemiMinorConfidence1;
SemiMajorOrientation = SemiMajorOrientation1;
Altitude = Altitude1;
Heading = Heading1;
HeadingConfidence = HeadingConfidence1;
Speed = Speed1;
SpeedConfidence = SpeedConfidence1;
VehicleLength = VehicleLength1;
VehicleWidth = VehicleWidth1;
LongAcceleration = LongAcceleration1;
LongAccelerationConfidence = LongAccelerationConfidence1;
YawRate = YawRate1;
YawRateConfidence = YawRateConfidence1;
VehicleRole = double(VehicleRole1);

% Insert a NaN if the bit mask indicates that the VehicleRole is not
% present
if bitget(ContainerMask1, 8) == 1
   VehicleRole = NaN;
end

== matlab function MessageUnpack/ParseICLCM ==
  data: MessageID output double; MessageID1 input double; StationID output double; ContainerMask output double; RearAxleLocation output double; ControllerType output double; ResponseTimeConstant output double; ResponseTimeDelay output double; TargetLongAcceleration output double; TimeHeadway output double; CruiseSpeed output double; LowFrequencyMask output double; ParticipantsReady output double; StartPlatoon output double; EndOfScenario output double; MioID output double; MioRange output double; MioBearing output double; MioRangeRate output double; Lane output double; ForwardID output double; BackwardID output double; AcknowledgmentFlag output double; MergeRequest output double; SafeToMerge output double; Flag output double; FlagTail output double; FlagHead output double; PlatoonID output double; DistanceTravelledInCz output double; Intention output double; Counter output double; StationID1 input double; ContainerMask1 input double; RearAxleLocation1 input double; ControllerType1 input double; ResponseTimeConstant1 input double; ResponseTimeDelay1 input double; TargetLongAcceleration1 input double; TimeHeadway1 input double; CruiseSpeed1 input double; LowFrequencyMask1 input double; ParticipantsReady1 input double; StartPlatoon1 input double; EndOfScenario1 input double; MioID1 input double; MioRange1 input double; MioBearing1 input double; MioRangeRate1 input double; Lane1 input double; ForwardID1 input double; BackwardID1 input double; AcknowledgmentFlag1 input double; MergeRequest1 input double; SafeToMerge1 input double; Flag1 input double; FlagTail1 input double; FlagHead1 input double; PlatoonID1 input double; DistanceTravelledInCz1 input double; Intention1 input double; Counter1 input double
function [MessageID, StationID, ContainerMask, RearAxleLocation, ControllerType, ResponseTimeConstant, ResponseTimeDelay, TargetLongAcceleration, TimeHeadway, CruiseSpeed, LowFrequencyMask, ParticipantsReady, StartPlatoon, EndOfScenario, MioID, MioRange, MioBearing, MioRangeRate, Lane, ForwardID, BackwardID, AcknowledgmentFlag, MergeRequest, SafeToMerge, Flag, FlagTail, FlagHead, PlatoonID, DistanceTravelledInCz, Intention, Counter] = parseICLCM(MessageID1, StationID1, ContainerMask1, RearAxleLocation1, ControllerType1, ResponseTimeConstant1, ResponseTimeDelay1, TargetLongAcceleration1, TimeHeadway1, CruiseSpeed1, LowFrequencyMask1, ParticipantsReady1, StartPlatoon1, EndOfScenario1, MioID1, MioRange1, MioBearing1, MioRangeRate1, Lane1, ForwardID1, BackwardID1, AcknowledgmentFlag1, MergeRequest1, SafeToMerge1, Flag1, FlagTail1, FlagHead1, PlatoonID1, DistanceTravelledInCz1, Intention1, Counter1)
%parseICLCM - Parses a local ICLCM.
MessageID = MessageID1;
StationID = StationID1;
ContainerMask = ContainerMask1;
RearAxleLocation = RearAxleLocation1;
ControllerType = ControllerType1;
ResponseTimeConstant = ResponseTimeConstant1;
ResponseTimeDelay = ResponseTimeDelay1;
TargetLongAcceleration = TargetLongAcceleration1;
TimeHeadway = TimeHeadway1;
CruiseSpeed = CruiseSpeed1;
LowFrequencyMask = LowFrequencyMask1;
ParticipantsReady = ParticipantsReady1;
StartPlatoon = StartPlatoon1;
EndOfScenario = EndOfScenario1;
MioID = MioID1;
MioRange = MioRange1;
MioBearing = MioBearing1;
MioRangeRate = MioRangeRate1;
Lane = Lane1;
ForwardID = ForwardID1;
BackwardID = BackwardID1;
AcknowledgmentFlag = AcknowledgmentFlag1;
MergeRequest = MergeRequest1;
SafeToMerge = SafeToMerge1;
Flag = Flag1;
FlagTail = FlagTail1;
FlagHead = FlagHead1;
PlatoonID = PlatoonID1;
DistanceTravelledInCz = DistanceTravelledInCz1;
Intention = Intention1;
Counter = Counter1;
